simulink model "a_LS_model"  (R2023b)
settings: Solver=VariableStepAuto  StartTime=0.0  StopTime=5  RelTol=1e-3
PreLoadFcn:
  | %% Model component value calculations with holder values.
  | clear;
  | disp('PreLoaded holder values run model to apply entered T&S values ')
  | 
  | Re = [1, 1]; % The DC resistance of the Voice coil [ohm].
  | 
  | Le = [1, 1]; % The voice coil inductance [H]
  | 
  | Mms = [1, 1]; % Mass of the coil and diaphragm [Kg]
  | 
  | Sd = [1, 1] * 1e-4; % Area of diaphragm [m^2]
  | 
  | Bl = [1, 1]; % The product of magnetic flux density i.e., Force Factor
  | 
  | Vb = [1, 1];
  | 
  | fs = [1, 1];
  | 
  | Qes = [1, 1];
  | 
  | Qms = [1, 1];
  | 
  | Qts = [1, 1];
  | 
  | SweepStart_W_S = 1;
  | SweepEnd_W_S = 1;
  | SweepDuration_W_S = 1;
  | FS = 44100;
  | Qb = 0.707; % Total quality factor
  | 
  | % Constants
  | c = 340; % Speed of sound in m/s
  | rho = 1.2; % Density of air [kg/m^3]
  | r=1; % Distance for farfield calculations
  | wOffset = 0; % Driver offset for fafield calculations not used in this version
  | tOffset = 0;
  | dt=1/FS; % Time step
  | for n = 1:2
  |     alpha(n) = (Qb^2 - Qts(n)^2) / Qts(n)^2;
  |     Rms(n) = (2 * pi * fs(n) * Mms(n)) / Qms(n);
  |     Cms(n) = 1 / (4 * pi^2 * fs(n)^2 * Mms(n));
  |     Vas(n) = rho * c * Sd(n)^2 * Cms(n);
  | end
  | 
  | QB = sqrt(alpha(1) + 1) * Qts; % Electroacoustics Lecture 4 page 21
  | 
  | for n = 1:2
  |     r = 0.1;
  |     Cab(n) = Vb(n) / (rho * c^2); % Box volume acoustic compliance
  |     a(n) = sqrt(Sd(n) / pi);
  |     a(n) = 0.85;
  | 
  |     % Zc(n) = ((rho * c) / Sd(n)) * c; % from grain42n
  |     Mad(n) = (8 * rho) / (5 * (pi^2) * a(n)); % Mad (acoustic mass)
  |     Mar(n) = rho * ((a(n) * r) / Sd(n)); % from grain42n
  |     Mad(n) = Mar(n);
  | 
  |     Ras(n) = (rho * c) / (pi * (a(n)^2)); % Ras (acoustic resistance), Beranek page 820/ grain42-page 19
  |     Lem(n) = Bl(n)^2 * Cms(n); % Lem (driver's compliane in electrical domain)
  |     Rem(n) = Bl(n)^2 / Rms(n); % Rem (driver's equivalent mechanical resistance)
  |     Cem(n) = Mms(n) / (Bl(n)^2); % Cem (driver's mass in Electrical domain) from grain41en
  | 
  | 
  | 
  |     Rer(n) = (Bl(n) / Sd(n))^2 * (1 / Ras(n)); % Rea (acoustical resistance) In Electrical
  |     Leb(n) = (Bl(n) / Sd(n))^2 * Cab(n); % Lea (acoustical complance) grain42-page 19
  | 
  |     Cer(n) = (Sd(n) / Bl(n))^2 * Mar(n); % (acoustical mass) in Electrical Domain (front)
  |     Ced(n) = (Sd(n) / Bl(n))^2 * Mad(n); %(acoustical mass) in Electrical Domain (back)
  | end
  | 
  | H_prev = complex(ones(512,1));
  | H_Bt = complex(zeros(512,1));
  | tweeterHz = double(0);
  | 
  | mex mexFilter.c
  | mex mexParaFilter.c
  | mex ohmsCalc.c
InitFcn:
  | Re = [str2double(get_param('a_LS_model/T&S Values', 'W_Re')), str2double(get_param('a_LS_model/T&S Values', 'T_Re'))]; % DC resistance of the Voice coil [ohm].
  | Le = [str2double(get_param('a_LS_model/T&S Values', 'W_Le')), str2double(get_param('a_LS_model/T&S Values', 'T_Le'))] * 1e-3; % Voice coil inductance [H]
  | Mms = [str2double(get_param('a_LS_model/T&S Values', 'W_Mms')), str2double(get_param('a_LS_model/T&S Values', 'T_Mms'))] * 1e-3; % Mass of the coil and diaphragm [Kg]
  | Sd = [str2double(get_param('a_LS_model/T&S Values', 'W_Sd')), str2double(get_param('a_LS_model/T&S Values', 'T_Sd'))] * 1e-4; % Area of diaphragm [m^2]
  | Bl = [str2double(get_param('a_LS_model/T&S Values', 'W_Bl')), str2double(get_param('a_LS_model/T&S Values', 'T_Bl'))]; % Magnetic flux density product (Force Factor)
  | Vb = [str2double(get_param('a_LS_model/T&S Values', 'Vb')), str2double(get_param('a_LS_model/T&S Values', 'Vb'))];
  | fs = [str2double(get_param('a_LS_model/T&S Values', 'W_fs')), str2double(get_param('a_LS_model/T&S Values', 'T_fs'))];
  | Cms = [str2double(get_param('a_LS_model/T&S Values', 'W_Cms')), str2double(get_param('a_LS_model/T&S Values', 'W_Cms'))];
  | Qes = [str2double(get_param('a_LS_model/T&S Values', 'W_Qes')), str2double(get_param('a_LS_model/T&S Values', 'T_Qes'))];
  | Qms = [str2double(get_param('a_LS_model/T&S Values', 'W_Qms')), str2double(get_param('a_LS_model/T&S Values', 'T_Qms'))];
  | Qts = [str2double(get_param('a_LS_model/T&S Values', 'W_Qts')), str2double(get_param('a_LS_model/T&S Values', 'T_Qts'))];
  | 
  | % Load additional parameters
  | SweepStart_W_S = str2double(get_param('a_LS_model/Subsystem4', 'SweepStart'));
  | SweepEnd_W_S = str2double(get_param('a_LS_model/Subsystem4', 'SweepStop'));
  | SweepDuration_W_S = str2double(get_param('a_LS_model/Subsystem4', 'SweepTime'));
  | 
  | 
  | FS = 44100;
  | 
  | % Constants
  | c = 343; % Speed of sound in m/s
  | rho = 1.2; % Density of air [kg/m^3]
  | wOffset = str2double(get_param('a_LS_model/Subsystem1', 'distW'));
  | tOffset = str2double(get_param('a_LS_model/Subsystem1', 'distT'));
  | dt=1/FS; %time step
  | 
  | Vas(1) = rho * c * Sd(1)^2 * Cms(1);
  | 
  | for n = 1:2
  |     if n == 1
  |      fsBx = fs(1) *(Vas(1)/Vb(1)+1)^(1/2);
  |      aV = Vas(1) / Vb(1);
  |      Qb(n) = Qts(n) * sqrt(1 + aV);
  |      Rms(n) = (2 * pi * fs(n) * Mms(n)) / Qms(n);
  |      Cms(n) = 1 / ((2 * pi * fs(n))^2 * Mms(n));
  |      CmsBx = 1 / ((2 * pi * fsBx)^2 * Mms(n));
  |      QmsBx =  (2*pi*fsBx*Mms(1))/Rms(1);
  |      RmsBx = (2 * pi * fsBx * Mms(n)) / (QmsBx);
  |     elseif n == 2
  | 
  |      Cms(n) = 1 / ((2 * pi * fs(n))^2 * Mms(n));
  |      Rms(n) = (2 * pi * fs(n) * Mms(n)) / Qms(n);
  |      Vas(n) = rho * c * Sd(n)^2 * Cms(n);
  | 
  |     end
  |    alpha(n) = (Qb^2 - Qts(n)^2) / Qts(n)^2;
  | 
  | end
  | 
  | QB = sqrt(alpha(1) + 1) * Qts; % Lecture 4 page 21
  | 
  | for n = 1:2
  |     r = 0.1;
  |     Cab(n) = Vb(n) / (rho * c^2); % Box volume acoustic compliance
  |     a(n) = sqrt(Sd(n) / pi);
  |     Mad(n) = (8 * rho) / (5 * (pi^2) * a(n)); % Mad (acoustic mass)
  |     Mar(n) = rho * ((a(n) * r) / Sd(n));
  |     Ras(n) = (rho * c) / (pi * (a(n)^2)); % Ras (acoustic resistance), Beranek page 820/ grain42-page 19
  | 
  |     Lem(n) = (Bl(n)^2) * (Cms(n)); %driver compliance in electrical Domain
  |     Rem(n) = (Bl(n)^2) / Rms(n); % mechanical resistance)
  |     Cem(n) = Mms(n) / (Bl(n)^2); % mass in electical domain)
  | 
  |     Leb(n) = (Bl(n) / Sd(n))^2 * Cab(n); % Lea (acoustical compliance)
  |     Rer(n) = (Bl(n) / Sd(n))^2 * 1 / Ras(n); % Rea (acoustical resistance)
  |     Cer(n) = (Sd(n) / Bl(n))^2 * Mar(n); % Cea (acoustical mass in electrical domain Front)
  |     Ced(n) = (Sd(n) / Bl(n))^2 * Mad(n); % (acoustical mass in ED back)
  | end
  | mex mexFilter.c
  | mex mexParaFilter.c
  | mex ohmsCalc.c
StartFcn:
  | %% Model Component Value Calculations beta
  | close all;
  | 
  | disp('Thiele and Small Parameters Loaded');
  | disp('Loudspeaker Simulation Running...');
  | 
  | % Load parameters from the mask
  | Box_plot_flag = get_param('a_LS_model/T&S Values', 'Box_Plot');
  | Combo_plot_flag = get_param('a_LS_model/T&S Values', 'DSP_Plot');
  | wImpedance_plot_flag = get_param('a_LS_model/T&S Values', 'wImpedance_Plot');
  | tImpedance_plot_flag = get_param('a_LS_model/T&S Values', 'tImpedance_Plot');
  | Re = [str2double(get_param('a_LS_model/T&S Values', 'W_Re')), str2double(get_param('a_LS_model/T&S Values', 'T_Re'))]; % DC resistance of the Voice coil [ohm].
  | Le = [str2double(get_param('a_LS_model/T&S Values', 'W_Le')), str2double(get_param('a_LS_model/T&S Values', 'T_Le'))] * 1e-3; % Voice coil inductance [H]
  | Mms = [str2double(get_param('a_LS_model/T&S Values', 'W_Mms')), str2double(get_param('a_LS_model/T&S Values', 'T_Mms'))] * 1e-3; % Mass of the coil and diaphragm [Kg]
  | Sd = [str2double(get_param('a_LS_model/T&S Values', 'W_Sd')), str2double(get_param('a_LS_model/T&S Values', 'T_Sd'))] * 1e-4; % Area of diaphragm [m^2]
  | Bl = [str2double(get_param('a_LS_model/T&S Values', 'W_Bl')), str2double(get_param('a_LS_model/T&S Values', 'T_Bl'))]; % Magnetic flux density product (Force Factor)
  | Vb = [str2double(get_param('a_LS_model/T&S Values', 'Vb')), str2double(get_param('a_LS_model/T&S Values', 'Vb'))];
  | fs = [str2double(get_param('a_LS_model/T&S Values', 'W_fs')), str2double(get_param('a_LS_model/T&S Values', 'T_fs'))];
  | Cms = [str2double(get_param('a_LS_model/T&S Values', 'W_Cms')), str2double(get_param('a_LS_model/T&S Values', 'W_Cms'))];
  | Qes = [str2double(get_param('a_LS_model/T&S Values', 'W_Qes')), str2double(get_param('a_LS_model/T&S Values', 'T_Qes'))];
  | Qms = [str2double(get_param('a_LS_model/T&S Values', 'W_Qms')), str2double(get_param('a_LS_model/T&S Values', 'T_Qms'))];
  | Qts = [str2double(get_param('a_LS_model/T&S Values', 'W_Qts')), str2double(get_param('a_LS_model/T&S Values', 'T_Qts'))];
  | 
  | % Load additional parameters
  | SweepStart_W_S = str2double(get_param('a_LS_model/Subsystem4', 'SweepStart'));
  | SweepEnd_W_S = str2double(get_param('a_LS_model/Subsystem4', 'SweepStop'));
  | SweepDuration_W_S = str2double(get_param('a_LS_model/Subsystem4', 'SweepTime'));
  | 
  | figSaveFolder = get_param('a_LS_model/Teensy Script', 'figSaveFolder');
  | 
  | FS = 44100;
  | 
  | % Constants
  | c = 343; % Speed of sound in m/s
  | rho = 1.2; % Density of air [kg/m^3]
  | wOffset = str2double(get_param('a_LS_model/Subsystem1', 'distW'));
  | tOffset = str2double(get_param('a_LS_model/Subsystem1', 'distT'));
  | dt=1/FS; %time step
  | 
  | Vas(1) = rho * c * Sd(1)^2 * Cms(1);
  | 
  | for n = 1:2
  |     if n == 1
  |      fsBx = fs(1) *(Vas(1)/Vb(1)+1)^(1/2);
  |      aV = Vas(1) / Vb(1);
  |      Qb(n) = Qts(n) * sqrt(1 + aV);
  |      Rms(n) = (2 * pi * fs(n) * Mms(n)) / Qms(n);
  |      Cms(n) = 1 / ((2 * pi * fs(n))^2 * Mms(n));
  |      CmsBx = 1 / ((2 * pi * fsBx)^2 * Mms(n));
  |      QmsBx =  (2*pi*fsBx*Mms(1))/Rms(1);
  |      RmsBx = (2 * pi * fsBx * Mms(n)) / (QmsBx);
  |     elseif n == 2
  | 
  |      Cms(n) = 1 / ((2 * pi * fs(n))^2 * Mms(n));
  |      Rms(n) = (2 * pi * fs(n) * Mms(n)) / Qms(n);
  |      Vas(n) = rho * c * Sd(n)^2 * Cms(n);
  | 
  |     end
  |    alpha(n) = (Qb^2 - Qts(n)^2) / Qts(n)^2;
  | 
  | end
  | 
  | QB = sqrt(alpha(1) + 1) * Qts; % Lecture 4 page 21
  | 
  | for n = 1:2
  |     r = 0.1;
  |     Cab(n) = Vb(n) / (rho * c^2); % Box volume acoustic compliance
  |     a(n) = sqrt(Sd(n) / pi);
  |     Mad(n) = (8 * rho) / (5 * (pi^2) * a(n)); % Mad (acoustic mass)
  |     Mar(n) = rho * ((a(n) * r) / Sd(n));
  |     Ras(n) = (rho * c) / (pi * (a(n)^2)); % Ras (acoustic resistance), Beranek page 820/ grain42-page 19
  | 
  |     Lem(n) = (Bl(n)^2) * (Cms(n)); %driver compliance in electrical domain
  |     Rem(n) = (Bl(n)^2) / Rms(n); % mechanical resistance in ED
  |     Cem(n) = Mms(n) / (Bl(n)^2); %moving mass in ED
  | 
  |     Leb(n) = (Bl(n) / Sd(n))^2 * Cab(n); % Lea (acoustical compliance in ED)
  |     Rer(n) = (Bl(n) / Sd(n))^2 * 1 / Ras(n); % Rea (acoustical resistance)
  |     Cer(n) = (Sd(n) / Bl(n))^2 * Mar(n); % (acoustical mass in ED front)
  |     Ced(n) = (Sd(n) / Bl(n))^2 * Mad(n); % (acoustical mass in ED back)
  | end
  | 
  | % Low-end box response plotting
  | for n = 1:2
  |     Cas(n) = Vas(n) / (rho * c^2);
  |     W0(n) = 1 / (sqrt((Mms(n)) / Sd(n)^2 * ((Cas(n) * Cab(n)) / (Cas(n) + Cab(n)))));
  |     f = 1:512;
  |     w = 2 * pi * f;
  |     k = w / c;
  | 
  |     if strcmp(Box_plot_flag, 'on')
  |         Hb = w.^2 ./ (w.^2 - (W0(1)^2) - 1j * (W0(1) / Qb(1)) * w);
  |         figure(3);
  |         semilogx(f, 20 * log10(abs(Hb)), 'r-', 'LineWidth', 2, 'DisplayName', 'Current');
  |         hold on;
  | 
  |         legend('show', 'Location', 'southeast');
  |         grid on;
  |         hold off;
  |         ylabel('Magnitude [dB]');
  |         xlim([20 600]);
  |         ylim([-20 5]);
  |         title('Low-end box response');
  |         xticks([20 62.5 125 250 500]);
  |         xticklabels({'20', '62.5', '125', '250', '500'});
  |         xlabel('Frequency Hz');
  | 
  |         if strcmp(get_param('a_LS_model/Teensy Script', 'saveFigs'),"on")
  | 
  |           if ~exist(figSaveFolder, 'dir')
  | 
  |                mkdir(figSaveFolder);
  | 
  |           end
  |             saveas(gcf,fullfile(figSaveFolder,[figSaveFolder,'_boxResponse.png']));
  |         end
  | 
  |     end
  | end
  | 
  | % PARAMETRIC EQ
  | if strcmp(Combo_plot_flag, 'on')
  | 
  |     Hb = w.^2 ./ (w.^2 - (W0(1)^2) - 1j * (W0(1) / Qb(1)) * w);
  | 
  |     fs = 44100;
  |     Numband = 6;
  | 
  |     V0 = zeros(Numband, 1);
  |     V0_peq = zeros(Numband, 1);
  |     K = zeros(Numband, 1);
  |     fc = zeros(Numband, 1);
  |     BWp = zeros(Numband, 1);
  |     BW = zeros(Numband, 1);
  |     N = zeros(Numband, 1);
  |     w0 = zeros(Numband, 1);
  |     gain = zeros(Numband, 1);
  |     H = complex(ones(22500, 1));
  |     H_temp = complex(ones(22500, Numband));
  | 
  | % Load filter parameters
  | 
  | gain(1) = str2double(get_param('a_LS_model/Subsystem', 'GdB1'));
  | gain(2) = str2double(get_param('a_LS_model/Subsystem', 'GdB2'));
  | gain(3) = str2double(get_param('a_LS_model/Subsystem', 'GdB3'));
  | gain(4) = str2double(get_param('a_LS_model/Subsystem', 'GdB4'));
  | gain(5) = str2double(get_param('a_LS_model/Subsystem', 'GdB5'));
  | gain(6) = str2double(get_param('a_LS_model/Subsystem', 'GdB6'));
  | 
  | fc(1) = str2double(get_param('a_LS_model/Subsystem', 'FC1'));
  | fc(2) = str2double(get_param('a_LS_model/Subsystem', 'FC2'));
  | fc(3) = str2double(get_param('a_LS_model/Subsystem', 'FC3'));
  | fc(4) = str2double(get_param('a_LS_model/Subsystem', 'FC4'));
  | fc(5) = str2double(get_param('a_LS_model/Subsystem', 'FC5'));
  | fc(6) = str2double(get_param('a_LS_model/Subsystem', 'FC6'));
  | 
  | BWp(1) = str2double(get_param('a_LS_model/Subsystem', 'BW1'));
  | BWp(2) = str2double(get_param('a_LS_model/Subsystem', 'BW2'));
  | BWp(3) = str2double(get_param('a_LS_model/Subsystem', 'BW3'));
  | BWp(4) = str2double(get_param('a_LS_model/Subsystem', 'BW4'));
  | BWp(5) = str2double(get_param('a_LS_model/Subsystem', 'BW5'));
  | BWp(6) = str2double(get_param('a_LS_model/Subsystem', 'BW6'));
  | 
  | Filt=zeros(Numband,4);
  | b0=double(0);
  | b1=double(0);
  | b2=double(0);
  | a0=double(0);
  | a1=double(0);
  | a2=double(0);
  | 
  | for i=1:Numband
  | 
  | Filt(i,1)= gain(i);
  | Filt(i,2)=fc(i);
  | Filt(i,3)=BWp(i);
  | Filt(i,4)=BWp(i)*gain(i);
  | end
  | 
  | minFc=min(Filt(1:end,2));
  | maxFc=max(Filt(1:end,2));
  | 
  | 
  | for i=1:Numband
  | V0(i)= 10^(Filt(i,1)/20);%For shelving filters
  |     K(i)= tan ((pi*fc(i))/fs);
  | 
  |     V0_peq(i)=Filt(i,1);%For peaking filter
  |     w0(i) = Filt(i,2)/(fs/2);
  |     N=double(2);
  | 
  | 
  | 
  |     BW(i)=(Filt(i,2)*Filt(i,3))/100;%percentage of fc to Hz
  |     BW(i)=BW(i)/(fs/2);
  | 
  | end
  | 
  | [B,A] = designParamEQ(2,V0_peq',w0', BW','Orientation','row');
  | 
  | a0=1;
  | for i=1:Numband
  | 
  | 
  |    if Filt(i,2) ==minFc && V0(i)>0
  |       %Low Shelf Boost
  |       b0 = ((1)+(sqrt(2*V0(i))*K(i))+V0(i)*K(i)^2) / ((1)+(sqrt(2)*K(i))+K(i)^2);
  |       b1 = ((2)*(V0(i)*(K(i)^2)-1)) / ((1)+(sqrt(2)*K(i))+K(i)^2);
  |       b2 = ((1)-(sqrt(2*V0(i))*K(i))+V0(i)*K(i)^2) / ((1)+(sqrt(2)*K(i))+K(i)^2);
  |       a1 =  ((2)*((K(i)^2)-1)) / ((1)+(sqrt(2)*K(i))+K(i)^2);
  |       a2 = ((1)-sqrt(2)*K(i)+K(i)^2) / ((1)+(sqrt(2)*K(i))+K(i)^2);
  | 
  |       B(i,:)=[b0,b1,b2];
  |       A(i,:)=[a0,a1,a2];
  | 
  |    elseif Filt(i,2) == minFc && V0(i)<0
  |       %Low Shelf Cut
  | 
  |       b0=(V0(i)*(1+sqrt(2)*K(i)+K(i)^2)) / (V0(i)+sqrt(2*V0(i))*K(i)+K(i)^2);
  |       b1=(2*V0(i)*(K(i)^2-1)) / (V0(i)+sqrt(2*V0(i))*K(i)+K(i)^2);
  |       b2=(V0(i)*(1-sqrt(2)*K(i)+K(i)^2)) / (V0(i)+sqrt(2*V0(i))*K(i)+K(i)^2);
  |       a1=(2*(K(i)^2-V0(i))) / (V0(i)+sqrt(2*V0(i))*K(i)+K(i)^2);
  |       a2=(V0(i)-sqrt(2*V0(i))*K(i)+K(i)^2) / (V0(i)+sqrt(2*V0(i))*K(i)+K(i)^2);
  | 
  |       B(i,:)=[b0,b1,b2];
  |       A(i,:)=[a0,a1,a2];
  | 
  | 
  |    elseif Filt(i,2) ==maxFc && V0(i)>0
  |       % High Shelf Boost
  |       b0 = (V0(i)+sqrt(2*V0(i))*K(i)+K(i)^2) /(1+sqrt(2)*K(i)+K(i)^2);
  |       b1= (2*(K(i)^2-V0(i))) / (1+sqrt(2)*K(i)+K(i)^2);
  |       b2=  (V0(i)-sqrt(2*V0(i))*K(i)+K(i)^2) / (1+sqrt(2)*K(i)+K(i)^2);
  |       a1= (2*(K(i)^2-1)) / (1+(sqrt(2)*K(i))+K(i)^2);
  |       a2= (1-(sqrt(2)*K(i))+K(i)^2) / (1+(sqrt(2)*K(i))+K(i)^2);
  | 
  |       B(i,:)=[b0,b1,b2];
  |       A(i,:)=[a0,a1,a2];
  | 
  |     elseif Filt(i,2) == maxFc && V0(i)<0
  |        %High Shelf Cut
  | 
  |         b0=(V0(i)*(1+sqrt(2)*K(i)+K(i)^2)) / (1+sqrt(2*V0(i))*K(i)+V0(i)*K(i)^2);
  |         b1=(2*V0(i)*(K(i)^2-1)) / (1+sqrt(2*V0(i))*K(i)+V0(i)*K(i)^2);
  |         b2=(V0(i)*(1-sqrt(2)*K(i)+K(i)^2)) / (1+sqrt(2*V0(i))*K(i)+V0(i)*K(i)^2);
  |         a1=(2*(V0(i)*K(i)^2-1)) / (1+sqrt(2*V0(i))*K(i)+V0(i)*K(i)^2);
  |         a2=(1-sqrt(2*V0(i))*K(i)+V0(i)*K(i)^2) / (1+sqrt(2*V0(i))*K(i)+V0(i)*K(i)^2);
  | 
  |         B(i,:)=[b0,b1,b2];
  |         A(i,:)=[a0,a1,a2];
  | 
  |         end
  | end
  | 
  | H=complex(ones(22500));
  | for n=1:6
  | 
  | [H_temp(1:end,n),w] = freqz(B(n,1:end),A(n,1:end),22500);
  | 
  | H=H.*H_temp(1:end,n);
  | end
  | forestGreen = [34/255, 139/255, 34/255];
  | H_trunc=H(1:512);
  | H_combine=H_trunc.*Hb;
  | f=1:512;
  |         figure(4)
  |         semilogx(f, 20 * log10(abs(Hb)), 'r-', 'LineWidth', 2, 'DisplayName', 'Box');
  | 
  |         hold on
  |         semilogx(f, 20 * log10(abs(H_combine)),'Color',forestGreen,'LineStyle', '--', 'LineWidth', 2, 'DisplayName', 'Box & DSP');
  | 
  |         xlabel('Frequency (Hz)')
  |         ylabel('Magnitude (dB)')
  |         title('Magnitude Response')
  | 
  | 
  | legend('show', 'Location', 'southeast');
  | grid on
  | xlim([20 550])
  | ylim([-20 5])
  | title('Low end box and DSP combined response')
  | xticks([(20) 62.5 125 250 500 ])
  | xticklabels({'20','62.5','125','250','500'})
  | xlabel('Frequency Hz');
  | hold off
  | if strcmp(get_param('a_LS_model/Teensy Script', 'saveFigs'),"on")
  | 
  |     if ~exist(figSaveFolder, 'dir')
  | 
  |                mkdir(figSaveFolder);
  | 
  |     end
  | 
  |     saveas(gcf,fullfile(figSaveFolder,[figSaveFolder,'_boxAndDsp.png']));
  | 
  | end
  | 
  | end
  | 
  | %% IMPEDANCES
  | %Woofer
  | if strcmp(wImpedance_plot_flag, "on")
  | frq = logspace(log10(20), log10(20000), 512);
  | w = 2 * pi * frq;
  | 
  | 
  | %Empirical Le rise correction factor
  | %Various attempts for HF accuracy
  | %{
  | N=length(w);
  | ZL = 1j.*w.*Le(1);
  | 
  | D =  sum(log(w).^2) - ((1/N) * sum(log(w)))^2 + (N * (pi/2)^2);
  | a =  sum(log(abs(ZL)).*log(w)) -(1/N)*sum(log(abs(ZL))).*sum(log(w))...
  |     +(pi/2).* sum(angle(ZL));
  | n = (1/D)*a;
  | LN_K = (1/N) * (sum(log(abs(ZL))) - n *sum(log(w)));
  | K = (exp(LN_K));
  | Ls = K .* (w.^n-1) .* sin((n.*pi) / 2)*1e-3;
  | Rs = K .* (w.^n) .* cos((n.*pi) / 2);
  | %}
  | R2p = Re(1);
  | L2p = Le(1);
  | 
  | %Zemp = 1./((1./(1j .* w .* Le(1))) + (1./(R2p+(1j.*w.*L2p))));
  | %Zemp2 = (R2p.*1j.*w.*L2p)./(R2p+(1j.*w.*L2p));
  | Zemp3 = (1j * w .* Le(1)) + ((R2p*(1j*w.*L2p)) / (R2p+(1j*w.*L2p)));
  | Z_ElectricalW =  Re(1) + Zemp3;
  | 
  | %CZobel Network Impedance
  | R_ZobelW = Re(1)*1.25 ;
  | Ce_ZobelW = Le(1)/(R_ZobelW^2);
  | Z_ZobelW = R_ZobelW + (1./(1j*w*Ce_ZobelW));
  | 
  | %Mechanical Impedance
  | 
  | MmsBx = Mms(1) * ((1+ (Vas(1)/Vb(1))));
  | CemBx = MmsBx / (Bl(1)^2);
  | 
  | LemBx = (Bl(1)^2) * CmsBx;
  | ResWBx = Bl(1)^2/ RmsBx;
  | ZcWMBx = 1./(1j.*w.*CemBx);
  | ZlWMBx = 1j.*w.*LemBx;
  | 
  | 
  | ResW = Bl(1)^2/ Rms(1);
  | ZcWM = 1./(1j.*w.*Cem(1));
  | ZlWM = 1j.*w.*Lem(1);
  | 
  | Z_MechanicalW = (1./ResW) +(1./ZcWM) + (1./ZlWM);
  | 
  | Z_MechanicalWBx = (1./ResWBx) +(1./ZcWM) + (1./ZlWMBx);
  | 
  | %Total Zs
  | Z_TotalW = Z_ElectricalW + (1 ./ Z_MechanicalW);
  | 
  | Z_TotalWBx = Z_ElectricalW + (1 ./ Z_MechanicalWBx);
  | 
  | Z_TotalWZobel =  (Z_ZobelW.* Z_TotalW) ./ (Z_ZobelW + Z_TotalW);
  | 
  | 
  | %Plotting
  | figure(9)
  | subplot(2,1,1)
  | 
  | semilogx(frq, abs(Z_TotalW) , 'b', 'LineWidth', 1, 'DisplayName', 'Woofer Impedance without Zobel');
  | hold on
  | semilogx(frq, abs(Z_TotalWZobel) , 'r --', 'LineWidth', 1, 'DisplayName', 'Woofer Impedance with Zobel');
  | semilogx(frq, abs(Z_TotalWBx) , 'g --', 'LineWidth', 1, 'DisplayName', 'Woofer Impedance in box');
  | 
  | 
  | hold off
  | xlabel('Frequency (Hz)');
  | ylabel('Impedance (ohms)');
  | title(sprintf('Woofer Impedance.\n Zobel Resistor: %.2f Ohm Zobel Capacitor: %.2f μF', R_ZobelW, Ce_ZobelW*1e6));
  | 
  | legend('Location', 'Best');
  | xlim([min(frq) max(frq)])
  | xticks([20 50 100 200 500 1000 2000 5000 10000 20000]);
  | xticklabels({'20','50','100','200','500','1000','2000','5000','10000','20000'});
  | 
  | subplot(2,1,2)
  | 
  | semilogx(frq, angle(Z_TotalW)*180/pi, 'r', 'LineWidth', 1, 'DisplayName', 'Woofer Phase');
  | 
  | xlabel('Frequency (Hz)');
  | ylabel('Angle (deg)');
  | title('Woofer Phase');
  | legend('Location', 'Best');
  | xlim([min(frq) max(frq)])
  | ylim([min(angle(Z_TotalW)*180/pi) max(angle(Z_TotalW)*180/pi)])
  | xticks([20 50 100 200 500 1000 2000 5000 10000 20000]);
  | 
  | if strcmp(get_param('a_LS_model/Teensy Script', 'saveFigs'),"on")
  | 
  |     if ~exist(figSaveFolder, 'dir')
  | 
  |                mkdir(figSaveFolder);
  | 
  |     end
  | 
  |     saveas(gcf,fullfile(figSaveFolder,[figSaveFolder,'_wooferImpedance.png']));
  | 
  | end
  | 
  | end
  | 
  | % Tweeter Impedance
  | if strcmp(tImpedance_plot_flag, "on")
  | 
  | %Zobel Network Impedance
  | R_ZobelT = Re(2)*1.25 ;
  | Ce_ZobelT = Le(2)/(R_ZobelT^2);
  | 
  | Z_ZobelT = R_ZobelT + (1./(1j*w*Ce_ZobelT));
  | 
  | %Empirical Electrical Impedance
  | %{
  | ZL = 1j.*w.*Le(2);
  | D =  sum(log(w).^2) - ((1/N) * sum(log(w)))^2 + (N * (pi/2)^2);
  | a =  sum(log(abs(ZL)).*log(w)) -(1/N)*sum(log(abs(ZL))).*sum(log(w))...
  |     +(pi/2).* sum(angle(ZL));
  | n = (1/D)*a;
  | LN_K = (1/N) * (sum(log(abs(ZL))) - n *sum(log(w)));
  | K = (exp(LN_K));
  | 
  | Ls=K.*(w.^n-1).*sin((n.*pi)/2);
  | Rs=K.*(w.^n).*cos((n.*pi)/2);
  | %}
  | R2p = Re(2);
  | L2p = Le(2);
  | Zemp = 1./((1./(1j .* w .* Le(2))) + (1./(R2p+(1j.*w.*L2p))));
  | Z_ElectricalT =  Re(2) + Zemp;
  | 
  | 
  | %Mechanical Impedance
  | ResT = Bl(2)^2/ Rms(2);
  | ZcTM = 1./(1j*w*Cem(2));
  | ZlTM = 1j*w*Lem(2);
  | 
  | Z_MechanicalT = (1./ResT) +(1./ZcTM) + (1./ZlTM);
  | 
  | %Total impedance with/without Zobel network
  | 
  | Z_TotalT =  Z_ElectricalT + (1 ./ Z_MechanicalT) ;
  | Z_TotalTZobel =  (Z_ZobelT.* Z_TotalT) ./ (Z_ZobelT + Z_TotalT);
  | 
  | %Impedances for Tweeter
  | figure(10)
  | subplot(2,1,1)
  | 
  | semilogx(frq, abs(Z_TotalT) , 'b', 'LineWidth', 1, 'DisplayName', 'Tweeter Impedance');
  | hold on
  | semilogx(frq, abs(Z_TotalTZobel) , 'r--', 'LineWidth', 1, 'DisplayName', 'Tweeter Impedance with Zobel');
  | hold off
  | 
  | xlabel('Frequency (Hz)');
  | ylabel('Impedance (ohms)');
  | title(sprintf('Tweeter Impedance.\n Zobel Resistor: %.2f Ohm Zobel Capacitor: %.2f μF', R_ZobelT, Ce_ZobelT*1e6));
  | legend('Location', 'Best');
  | xlim([min(frq) max(frq)])
  | ylim([min(abs(Z_TotalTZobel)-2) max(abs(Z_TotalT)+2)])
  | 
  | 
  | xticks([20 50 100 200 500 1000 2000 5000 10000 20000]);
  | xticklabels({'20','50','100','200','500','1000','2000','5000','10000','20000'});
  | xlim([min(frq) max(frq)]);
  | subplot(2,1,2)
  | semilogx(frq, angle(Z_TotalT)*180/pi, 'r', 'LineWidth', 1, 'DisplayName', 'Tweeter Phase');
  | 
  | xlabel('Frequency (Hz)');
  | ylabel('Angle (deg)');
  | title('Tweeter Phase');
  | legend('Location', 'Best');
  | xlim([min(frq) max(frq)])
  | ylim([min(angle(Z_TotalT)*180/pi) max(angle(Z_TotalT)*180/pi)])
  | xticks([20 50 100 200 500 1000 2000 5000 10000 20000]);
  | xticklabels({'20','50','100','200','500','1000','2000','5000','10000','20000'});
  | 
  | if strcmp(get_param('a_LS_model/Teensy Script', 'saveFigs'),"on")
  | 
  |     if ~exist(figSaveFolder, 'dir')
  | 
  |                mkdir(figSaveFolder);
  | 
  |     end
  | 
  |     saveas(gcf,fullfile(figSaveFolder,[figSaveFolder,'_tweeterImpedance.png']));
  | 
  | end
  | end
StopFcn:
  | disp('Simulation Ended')
undefined symbols (not defined in the file): Ced, Cem, Cer, Leb, Lem, Rem
libraries: fl_lib x32, nesl_utility x12, dspsrcs4 x1
(part 1 of 2)
settings Model: SimulationMode=accelerator  Creator=Jamie  LastModifiedBy=jamie
settings HardwareCC: ProdBitPerLong=64  ProdHWDeviceType=Intel->x86-64 (Mac OS X)

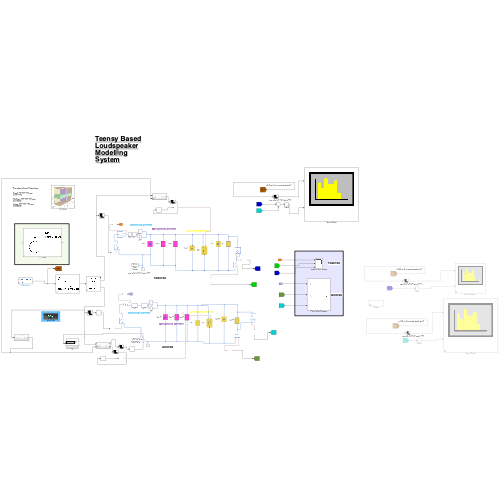
[thumbnail: Simulink's stored preview of the top-level diagram]
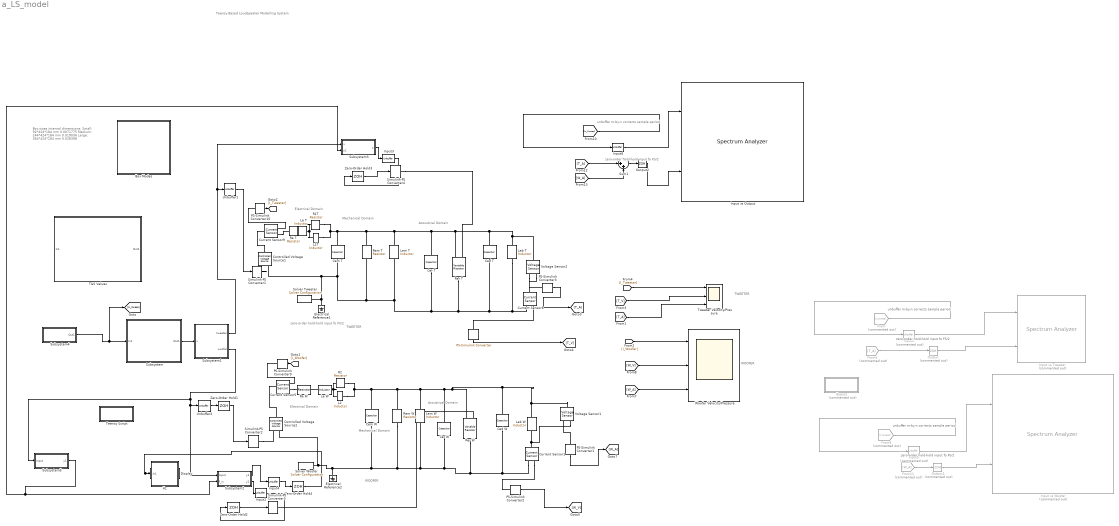
== system a_LS_model ==
  note: Teensy Based Loudspeaker Modelling System
  note: Box sizes internal dimensions:
      |
      | Small: 92*424*184 mm
      | 0.0071775
      |
      | Medium: 244*424*184 mm
      | 0.019036
      |
      | Large: 364*424*184 mm
      | 0.028398
  note: Electrical Domain
  note: Mechanical Domain
  note: Mechanical Domain
  note: WOOFER
  note: WOOFER
  note: unbuffer m-by-n corrects sample period
  note: TWEETER
  note: zero-order hold-hold input fo FS/2
  note: zero-order hold-hold input fo FS/2
  note: TWEETER
  note: Electrical Domain
  note: Acoustical Domain
  note: zero-order hold-hold input fo FS/2
  note: unbuffer m-by-n corrects sample period
  note: zero-order hold-hold input fo FS/2
  note: unbuffer m-by-n corrects sample period
  note: Acoustical Domain
  " " : nesl_utility/PS-Simulink Converter  PhysicalDomain=network_engine_domain  SubClassName=ps_output  LeftPortType=input  RightPortType=output  PseudoPeriodic=off  Frequencies=[]  VectorFormat=1-D array  Unit=1  AffineConversion=off
  Box Modes : Subsystem  mask{depth=244, height=424, width=184, vol=0.019036, boxFlag=on}
      mask prompts: depth "Depth (mm)"; height "Height (mm)"; width "Width (mm)"; vol "Volume (m^3)"; boxFlag "Calculate box modes on run (check this if using auto fig save feature)"
      mask DialogControl Control2 Prompt: Calculate volume
      mask DialogControl Control2 Callback:
      | depth= str2double(get_param('a_LS_model/Box Modes', 'depth'))*1e-3;
      | height = str2double(get_param('a_LS_model/Box Modes', 'height'))*1e-3;
      | width = str2double(get_param('a_LS_model/Box Modes', 'width'))*1e-3;
      | 
      | vol = depth*height*width;
      | 
      | set_param('a_LS_model/Box Modes','vol',num2str(vol));
      mask DialogControl Control4 Prompt: Show Box Modes
      mask DialogControl Control4 Callback:
      | depth= str2double(get_param('a_LS_model/Box Modes', 'depth'))*1e-3;
      | height = str2double(get_param('a_LS_model/Box Modes', 'height'))*1e-3;
      | width = str2double(get_param('a_LS_model/Box Modes', 'width'))*1e-3;
      | numberOfModes = 8;
      | rowNames = cell(numberOfModes,1);
      | 
      | 
      | 
      | 
      |     c = 343;
      | 
      | 
      | 
      | 
      |     depthModes = ones(numberOfModes,1);
      |     heightModes = ones(numberOfModes,1);
      |     widthModes = ones(numberOfModes,1);
      | 
      |     for i=1:numberOfModes
      | 
      |         depthModes(i)= floor((c/(2*depth))*i);
      |         heightModes(i) = floor((c/(2*height))*i);
      |         widthModes (i) = floor((c/(2*width))*i);
      | 
      |     end
      | 
      | 
      |     cNames = {'Depth'; 'Height'; 'Width'};
      | 
      | 
      |     modes = [depthModes, heightModes, widthModes];
      |     found=zeros(size(modes));
      |     toFind=double(0);
      | 
      |     %loop through matrix to find duplicates
      | 
      |     for m=1:3
      |         for j =1:numberOfModes
      |             toFind=modes(j,m);
      |             for n=1:3
      |                 for i=int8(1):numberOfModes
      |                     if modes(i, n) == toFind && (i ~= j && n ~= m)
      |                         found(i,n) = modes(i,n);
      | 
      |                     end
      |                 end
      |             end
      | 
      |         end
      | 
      |     end
      | 
      | 
      |     for i =int8(1):numberOfModes
      | 
      |         rowNames {i} = sprintf('Mode %d\n (Hz)',i);
      | 
      |     end
      | 
      | 
      | 
      | 
      |     figure(12)
      |     panel1 = uipanel('Title', 'Box Modes', 'TitlePosition','centertop','Position', [0.05, 0.05, 0.5, 0.9], 'FontSize', 18,'BackgroundColor', '#FFFDD0');
      |     panel2 = uipanel('Title', 'Duplicate Modes','TitlePosition','centertop', 'Position', [0.55, 0.05, 0.4, 0.9],'FontSize', 18, 'BackgroundColor', '#FFFDD0');
      | 
      |     uitable(panel1,"Data",modes, "ColumnName",cNames, 'RowName', rowNames,'Units', 'normalized','FontSize', 18);
      | 
      | 
      | 
      |     data = found;
      | 
      |     uitable(panel2, 'Data', data, "ColumnName",cNames,'RowName',rowNames, 'Units', 'normalized','FontSize', 18);
      | 
      |    set(gcf,'Position',[10 10 1000 400])
      mask DialogControl Control3 Prompt: To use this box volume in the model copy and paste it to the T&S Parameters block
      mask Display: image('modes.png'); % Use "Edit Image" on toolstrip to change.
  Bypass : Subsystem  Commented=on  mask{bypass=off}
      mask prompts: bypass "Bypass crossover/delay (for driver response)"
      mask DialogControl DescTextVar Prompt: This bypasses the crossover/delay/gain so the tweeter and woofer responses can be seen across full frequency band
  Ced T : fl_lib/Electrical/Electrical Elements/Capacitor  c=Ced(2) F  r=0 Ohm  g=0 1/Ohm  i_specify=off  i_priority=High  i=0 A  i_nominal_specify=off  i_nominal_unit=A  i_nominal_value=1  v_specify=off  v_priority=High  v=0 V  v_nominal_specify=off  v_nominal_unit=V  v_nominal_value=1  vc_specify=off  vc_priority=High  vc=0 V  vc_nominal_specify=off  vc_nominal_unit=V  vc_nominal_value=1
  Ced W : fl_lib/Electrical/Electrical Elements/Capacitor  c=Cer(1) F  r=0 Ohm  g=0 1/Ohm  i_specify=off  i_priority=High  i=0 A  i_nominal_specify=off  i_nominal_unit=A  i_nominal_value=1  v_specify=off  v_priority=High  v=0 V  v_nominal_specify=off  v_nominal_unit=V  v_nominal_value=1  vc_specify=off  vc_priority=High  vc=0 V  vc_nominal_specify=off  vc_nominal_unit=V  vc_nominal_value=1
  Cem T : fl_lib/Electrical/Electrical Elements/Capacitor  c=Cem(2) mF  r=0 Ohm  g=0 1/Ohm  i_specify=off  i_priority=High  i=0 A  i_nominal_specify=off  i_nominal_unit=A  i_nominal_value=1  v_specify=off  v_priority=High  v=0 V  v_nominal_specify=off  v_nominal_unit=V  v_nominal_value=1  vc_specify=off  vc_priority=High  vc=0 V  vc_nominal_specify=off  vc_nominal_unit=V  vc_nominal_value=1
  Cem W : fl_lib/Electrical/Electrical Elements/Capacitor  c=Cem(1) mF  r=0 Ohm  g=0 1/Ohm  i_specify=off  i_priority=High  i=0 A  i_nominal_specify=off  i_nominal_unit=A  i_nominal_value=1  v_specify=off  v_priority=High  v=0 V  v_nominal_specify=off  v_nominal_unit=V  v_nominal_value=1  vc_specify=off  vc_priority=High  vc=0 V  vc_nominal_specify=off  vc_nominal_unit=V  vc_nominal_value=1
  Cer T : fl_lib/Electrical/Electrical Elements/Capacitor  c=Cer(2) F  r=0 Ohm  g=0 1/Ohm  i_specify=off  i_priority=High  i=0 A  i_nominal_specify=off  i_nominal_unit=A  i_nominal_value=1  v_specify=off  v_priority=High  v=0 V  v_nominal_specify=off  v_nominal_unit=V  v_nominal_value=1  vc_specify=off  vc_priority=High  vc=0 V  vc_nominal_specify=off  vc_nominal_unit=V  vc_nominal_value=1
  Cer W : fl_lib/Electrical/Electrical Elements/Capacitor  c=Cer(1) F  r=0 Ohm  g=0 1/Ohm  i_specify=off  i_priority=High  i=0 A  i_nominal_specify=off  i_nominal_unit=A  i_nominal_value=1  v_specify=off  v_priority=High  v=0 V  v_nominal_specify=off  v_nominal_unit=V  v_nominal_value=1  vc_specify=off  vc_priority=High  vc=0 V  vc_nominal_specify=off  vc_nominal_unit=V  vc_nominal_value=1
  Controlled Voltage Source1 : fl_lib/Electrical/Electrical Sources/Controlled Voltage Source
  Controlled Voltage Source2 : fl_lib/Electrical/Electrical Sources/Controlled Voltage Source
  Current Sensor{1,5,8..9} (4 alike) : fl_lib/Electrical/Electrical Sensors/Current Sensor
  Display : Display
  Electrical Reference1 : fl_lib/Electrical/Electrical Elements/Electrical Reference
  Electrical Reference2 : fl_lib/Electrical/Electrical Elements/Electrical Reference
  From : From  Commented=on  GotoTag=In_Sweep
  From11 : From  Commented=on  GotoTag=W_A
  From5 : From  Commented=on  GotoTag=T_A
  From9 : From  Commented=on  GotoTag=In_Sweep
  Hz : Subsystem
  Input vs Output : SpectrumAnalyzer  NumInputPorts=2  WindowPosition=[1.000000,76.000000,1680.000000,922.000000,]  ScopeFrameLocation=window  Method=Welch  SampleRate=48000  PlotAsTwoSidedSpectrum=off  FrequencyScale=Log  AxesScaling=Manual  FrequencySpan=Start and stop frequencies  StartFrequency=4000  StopFrequency=20e3  AveragingMethod=Exponential  ForgettingFactor=0.4  FrequencyOffset=[500]  PlotNormalTrace=off  PlotMaxHoldTrace=on  YLimits=[-40.3301749,41.95165102]  ShowLegend=on
      settings: OpenAtSimulationStart=off
  "Input vs Tweeter  " : SpectrumAnalyzer  Commented=on  NumInputPorts=2  WindowPosition=[1.000000,76.000000,1680.000000,922.000000,]  ScopeFrameLocation=window  Method=Welch  SampleRate=48000  PlotAsTwoSidedSpectrum=off  FrequencyScale=Log  AxesScaling=Manual  FrequencySpan=Start and stop frequencies  StartFrequency=4000  StopFrequency=20e3  AveragingMethod=Exponential  ForgettingFactor=0.4  PlotNormalTrace=off  PlotMaxHoldTrace=on  YLimits=[-235.56274436,46.83172767]  ShowLegend=on
      settings: OpenAtSimulationStart=off
  Input vs Woofer : SpectrumAnalyzer  Commented=on  NumInputPorts=2  WindowPosition=[1.000000,76.000000,1680.000000,922.000000,]  ScopeFrameLocation=window  Method=Welch  SampleRate=48000  PlotAsTwoSidedSpectrum=off  FrequencyScale=Log  AxesScaling=Manual  FrequencySpan=Start and stop frequencies  StartFrequency=4000  StopFrequency=20e3  AveragingMethod=Exponential  ForgettingFactor=0.4  FrequencyOffset=[500]  PlotNormalTrace=off  PlotMaxHoldTrace=on  YLimits=[-193.2947565,31.72728743]  ShowLegend=on
      settings: OpenAtSimulationStart=off
  Input1 : Unbuffer  Commented=on
  Input{2..4,6} (4 alike) : Unbuffer
  Input5 : Unbuffer  Commented=on
  L1T : fl_lib/Electrical/Electrical Elements/Inductor  l=Le(2) H  r=0 Ohm  g=0 1/Ohm  i_specify=off  i_priority=High  i=0 A  i_nominal_specify=off  i_nominal_unit=A  i_nominal_value=1  v_specify=off  v_priority=High  v=0 V  v_nominal_specify=off  v_nominal_unit=V  v_nominal_value=1  i_L_specify=off  i_L_priority=High  i_L=0 A  i_L_nominal_specify=off  i_L_nominal_unit=A  i_L_nominal_value=1
  L2 : fl_lib/Electrical/Electrical Elements/Inductor  l=Le(1) H  r=0 Ohm  g=0 1/Ohm  i_specify=off  i_priority=High  i=0 A  i_nominal_specify=off  i_nominal_unit=A  i_nominal_value=1  v_specify=off  v_priority=High  v=0 V  v_nominal_specify=off  v_nominal_unit=V  v_nominal_value=1  i_L_specify=off  i_L_priority=High  i_L=0 A  i_L_nominal_specify=off  i_L_nominal_unit=A  i_L_nominal_value=1
  Le T : fl_lib/Electrical/Electrical Elements/Inductor  l=Le(2) H  r=0 Ohm  g=0 1/Ohm  i_specify=off  i_priority=High  i=0 A  i_nominal_specify=off  i_nominal_unit=A  i_nominal_value=1  v_specify=off  v_priority=High  v=0 V  v_nominal_specify=off  v_nominal_unit=V  v_nominal_value=1  i_L_specify=off  i_L_priority=High  i_L=0 A  i_L_nominal_specify=off  i_L_nominal_unit=A  i_L_nominal_value=1
  Le W : fl_lib/Electrical/Electrical Elements/Inductor  l=Le(1) H  r=0 Ohm  g=0 1/Ohm  i_specify=off  i_priority=High  i=0 A  i_nominal_specify=off  i_nominal_unit=A  i_nominal_value=1  v_specify=off  v_priority=High  v=0 V  v_nominal_specify=off  v_nominal_unit=V  v_nominal_value=1  i_L_specify=off  i_L_priority=High  i_L=0 A  i_L_nominal_specify=off  i_L_nominal_unit=A  i_L_nominal_value=1
  Leb T : fl_lib/Electrical/Electrical Elements/Inductor  l=Leb(2) mH  r=0 Ohm  g=0 1/Ohm  i_specify=off  i_priority=High  i=0 A  i_nominal_specify=off  i_nominal_unit=A  i_nominal_value=1  v_specify=off  v_priority=High  v=0 V  v_nominal_specify=off  v_nominal_unit=V  v_nominal_value=1  i_L_specify=off  i_L_priority=High  i_L=0 A  i_L_nominal_specify=off  i_L_nominal_unit=A  i_L_nominal_value=1
  Leb W : fl_lib/Electrical/Electrical Elements/Inductor  l=Leb(1) H  r=0 Ohm  g=0 1/Ohm  i_specify=off  i_priority=High  i=0 A  i_nominal_specify=off  i_nominal_unit=A  i_nominal_value=1  v_specify=off  v_priority=High  v=0 V  v_nominal_specify=off  v_nominal_unit=V  v_nominal_value=1  i_L_specify=off  i_L_priority=High  i_L=0 A  i_L_nominal_specify=off  i_L_nominal_unit=A  i_L_nominal_value=1
  Lem T : fl_lib/Electrical/Electrical Elements/Inductor  l=Lem(2) H  r=0 Ohm  g=0 1/Ohm  i_specify=off  i_priority=High  i=0 A  i_nominal_specify=off  i_nominal_unit=A  i_nominal_value=1  v_specify=off  v_priority=High  v=0 V  v_nominal_specify=off  v_nominal_unit=V  v_nominal_value=1  i_L_specify=off  i_L_priority=High  i_L=0 A  i_L_nominal_specify=off  i_L_nominal_unit=A  i_L_nominal_value=1
  Lem W : fl_lib/Electrical/Electrical Elements/Inductor  l=Lem(1) H  r=0 Ohm  g=0 1/Ohm  i_specify=off  i_priority=High  i=0 A  i_nominal_specify=off  i_nominal_unit=A  i_nominal_value=1  v_specify=off  v_priority=High  v=0 V  v_nominal_specify=off  v_nominal_unit=V  v_nominal_value=1  i_L_specify=off  i_L_priority=High  i_L=0 A  i_L_nominal_specify=off  i_L_nominal_unit=A  i_L_nominal_value=1
  Output : ZeroOrderHold  Commented=on  SampleTime=1/FS
  Output1 : ZeroOrderHold  Commented=on  SampleTime=1/FS
  Output2 : ZeroOrderHold  SampleTime=1/FS
  PS-Simulink Converter{1..3,9..10} (5 alike) : nesl_utility/PS-Simulink Converter  PhysicalDomain=network_engine_domain  SubClassName=ps_output  LeftPortType=input  RightPortType=output  PseudoPeriodic=off  Frequencies=[]  VectorFormat=1-D array  Unit=1  AffineConversion=off
  R1T : fl_lib/Electrical/Electrical Elements/Resistor  R=Re(2) Ohm  i_specify=off  i_priority=High  i=0 A  i_nominal_specify=off  i_nominal_unit=A  i_nominal_value=1  v_specify=off  v_priority=High  v=0 V  v_nominal_specify=off  v_nominal_unit=V  v_nominal_value=1
  R2 : fl_lib/Electrical/Electrical Elements/Resistor  R=Re(1) Ohm  i_specify=off  i_priority=High  i=0 A  i_nominal_specify=off  i_nominal_unit=A  i_nominal_value=1  v_specify=off  v_priority=High  v=0 V  v_nominal_specify=off  v_nominal_unit=V  v_nominal_value=1
  Re T : fl_lib/Electrical/Electrical Elements/Resistor  R=Re(2) Ohm  i_specify=off  i_priority=High  i=0 A  i_nominal_specify=off  i_nominal_unit=A  i_nominal_value=1  v_specify=off  v_priority=High  v=0 V  v_nominal_specify=off  v_nominal_unit=V  v_nominal_value=1
  Re W : fl_lib/Electrical/Electrical Elements/Resistor  R=Re(1) Ohm  i_specify=off  i_priority=High  i=0 A  i_nominal_specify=off  i_nominal_unit=A  i_nominal_value=1  v_specify=off  v_priority=High  v=0 V  v_nominal_specify=off  v_nominal_unit=V  v_nominal_value=1
  Rem T : fl_lib/Electrical/Electrical Elements/Resistor  R=Rem(2) Ohm  i_specify=off  i_priority=High  i=0 A  i_nominal_specify=off  i_nominal_unit=A  i_nominal_value=1  v_specify=off  v_priority=High  v=0 V  v_nominal_specify=off  v_nominal_unit=V  v_nominal_value=1
  Rem W : fl_lib/Electrical/Electrical Elements/Resistor  R=Rem(1) Ohm  i_specify=off  i_priority=High  i=0 A  i_nominal_specify=off  i_nominal_unit=A  i_nominal_value=1  v_specify=off  v_priority=High  v=0 V  v_nominal_specify=off  v_nominal_unit=V  v_nominal_value=1
  Rer T : fl_lib/Electrical/Electrical Elements/Variable Resistor  Rmin=0 Ohm  thermalEnable=false  thermal_mass=1 J/K  i_specify=off  i_priority=None  i=0 A  i_nominal_specify=off  i_nominal_unit=A  i_nominal_value=1  v_specify=off  v_priority=None  v=0 V  v_nominal_specify=off  v_nominal_unit=V  v_nominal_value=1  T_specify=off  T_priority=None  T=300 K  T_nominal_specify=off  T_nominal_unit=K  T_nominal_value=1
  Rer W : fl_lib/Electrical/Electrical Elements/Variable Resistor  Rmin=0 Ohm  thermalEnable=false  thermal_mass=1 J/K  i_specify=off  i_priority=None  i=0 A  i_nominal_specify=off  i_nominal_unit=A  i_nominal_value=1  v_specify=off  v_priority=None  v=0 V  v_nominal_specify=off  v_nominal_unit=V  v_nominal_value=1  T_specify=off  T_priority=None  T=300 K  T_nominal_specify=off  T_nominal_unit=K  T_nominal_value=1
  Simulink-PS Converter{1..4} (4 alike) : nesl_utility/Simulink-PS Converter  PhysicalDomain=network_engine_domain  SubClassName=ps_input  LeftPortType=input  RightPortType=output  PseudoPeriodic=off  Frequencies=[]  NoiseDistribution=none  NoiseParameters=[]  Unit=1  AffineConversion=off  FilteringAndDerivatives=zero  SimscapeFilterOrder=1  InputFilterTimeConstant=0.001  UdotUserProvided=1
  Solver Tweeter : nesl_utility/Solver Configuration  PhysicalDomain=network_engine_domain  SubClassName=solver  LeftPortType=input  RightPortType=generic  Tones=[]  Harmonics=[]  SimulateNoise=off  Profile=off  UseLocalSampling=off  EnableSwitchedLinearOptims=on  FrequencyDomain=off  UseCCode=off  RelTol=0.001  AbsTol=1e-06  MinStep=1e-09  ToWorkspace=off  RevertToSquareIcSolve=off  NumHomotopyIterations=100  PhasorMode=off  PhasorModeNumHarmonics=1  ConsistencySolver=NEWTON_FTOL  IndexReductionMethod=DerivativeReplacement  DoDC=off  ResidualTolerance=1e-09  ConsistencyTolSource=GLOBAL  ConsistencyAbsTol=0.001  ConsistencyRelTol=0.001  ConsistencyTolFactor=0.001  UseLocalSolver=off  LocalSolverChoice=NE_BACKWARD_EULER_ADVANCER  ResolveIndetEquations=on  FunctionEvalNumThread=1  LocalSolverSampleTime=0.001  DoFixedCost=off  MaxNonlinIter=3  MaxModeIter=2  ComputeImpulses=off  ImpulseIterations=2  LinearAlgebra=Sparse  LinearAlgebraNumThread=0  EquationFormulation=NE_TIME_EF  DelaysMemoryBudget=1024  AutomaticFiltering=on  FilteringTimeConstant=0.001  PartitionStorageMethod=AS_NEEDED  PartitionMemoryBudget=1024  PartitionMethod=FAST  MultibodyUseLocalSolver=off  MultibodyLocalSolverChoice=ODE1  MultibodyLocalSolverSampleTime=0.001
  "Solver Woofer " : nesl_utility/Solver Configuration  PhysicalDomain=network_engine_domain  SubClassName=solver  LeftPortType=input  RightPortType=generic  Tones=[]  Harmonics=[]  SimulateNoise=off  Profile=off  UseLocalSampling=off  EnableSwitchedLinearOptims=on  FrequencyDomain=off  UseCCode=off  RelTol=0.001  AbsTol=1e-06  MinStep=1e-09  ToWorkspace=off  RevertToSquareIcSolve=off  NumHomotopyIterations=100  PhasorMode=off  PhasorModeNumHarmonics=1  ConsistencySolver=NEWTON_FTOL  IndexReductionMethod=DerivativeReplacement  DoDC=off  ResidualTolerance=1e-09  ConsistencyTolSource=GLOBAL  ConsistencyAbsTol=0.001  ConsistencyRelTol=0.001  ConsistencyTolFactor=0.001  UseLocalSolver=off  LocalSolverChoice=NE_BACKWARD_EULER_ADVANCER  ResolveIndetEquations=on  FunctionEvalNumThread=1  LocalSolverSampleTime=0.001  DoFixedCost=off  MaxNonlinIter=3  MaxModeIter=2  ComputeImpulses=off  ImpulseIterations=2  LinearAlgebra=Sparse  LinearAlgebraNumThread=0  EquationFormulation=NE_TIME_EF  DelaysMemoryBudget=1024  AutomaticFiltering=on  FilteringTimeConstant=0.001  PartitionStorageMethod=AS_NEEDED  PartitionMemoryBudget=1024  PartitionMethod=FAST  MultibodyUseLocalSolver=off  MultibodyLocalSolverChoice=ODE1  MultibodyLocalSolverSampleTime=0.001
  Subsystem : Subsystem  mask{plotFlag=on, BW1=100.0, GdB1=2.9, FC1=78, BW2=78.150, GdB2=0.540, FC2=112, BW3=26.850, GdB3=0, FC3=3300, BW4=67.330, GdB4=0, FC4=2.000e+04, BW5=67.700, GdB5=0.13, FC5=180, BW6=89.550, GdB6=0.0, FC6=4000}
      mask prompts: plotFlag "Plot EQ response on run (needed for figure save function)"; BW1 "Band Width 1"; GdB1 "Gain 1"; FC1 "Center Frequency 1"; BW2 "Band Width 2"; GdB2 "Gain 2"; FC2 "Center Frequency 2"; BW3 "Band Width 3"; GdB3 "Gain 3"; FC3 "Center Frequency 3"; BW4 "Band Width 4"; GdB4 "Gain 4"; FC4 "Center Frequency 4"; BW5 "Band Width 5"; GdB5 "Gain 5"; FC5 "Center Frequency 5"; BW6 "Band Width 6"; GdB6 "Gain 6"; FC6 "Center Frequency 6"
      mask DialogControl DescTextVar Prompt: Highest and lowest fc will be shelving
      mask DialogControl Control2 Prompt: View EQ response
      mask DialogControl Control2 Callback:
      | fs =44100;
      | 
      | 
      | 
      | Numband = 6;
      | V0=zeros(Numband,1);
      | V0_peq=zeros(Numband,1);
      | K= zeros(Numband,1);
      | fc=zeros(Numband,1);
      | zeroLine=zeros(512,1);
      | BWp=zeros(Numband,1);
      | BW=zeros(Numband,1);
      | N=zeros(Numband,1);
      | w0=zeros(Numband,1);
      | H=complex(ones(512,1));
      | H_temp=complex(ones(512,Numband));
      | 
      | 
      | gain(1) = str2double(get_param('a_LS_model/Subsystem', 'GdB1'));
      | gain(2) = str2double(get_param('a_LS_model/Subsystem', 'GdB2'));
      | gain(3) = str2double(get_param('a_LS_model/Subsystem', 'GdB3'));
      | gain(4) = str2double(get_param('a_LS_model/Subsystem', 'GdB4'));
      | gain(5) = str2double(get_param('a_LS_model/Subsystem', 'GdB5'));
      | gain(6) = str2double(get_param('a_LS_model/Subsystem', 'GdB6'));
      | 
      | 
      | 
      | fc(1) = str2double(get_param('a_LS_model/Subsystem', 'FC1'));
      | fc(2) = str2double(get_param('a_LS_model/Subsystem', 'FC2'));
      | fc(3) = str2double(get_param('a_LS_model/Subsystem', 'FC3'));
      | fc(4) = str2double(get_param('a_LS_model/Subsystem', 'FC4'));
      | fc(5) = str2double(get_param('a_LS_model/Subsystem', 'FC5'));
      | fc(6) = str2double(get_param('a_LS_model/Subsystem', 'FC6'));
      | 
      | 
      | BWp(1) = str2double(get_param('a_LS_model/Subsystem', 'BW1'));
      | BWp(2) = str2double(get_param('a_LS_model/Subsystem', 'BW2'));
      | BWp(3) = str2double(get_param('a_LS_model/Subsystem', 'BW3'));
      | BWp(4) = str2double(get_param('a_LS_model/Subsystem', 'BW4'));
      | BWp(5) = str2double(get_param('a_LS_model/Subsystem', 'BW5'));
      | BWp(6) = str2double(get_param('a_LS_model/Subsystem', 'BW6'));
      | 
      | Filt=zeros(Numband,4);
      | b0=double(0);
      | b1=double(0);
      | b2=double(0);
      | a0=double(0);
      | a1=double(0);
      | a2=double(0);
      | 
      | for i=1:Numband
      | 
      | Filt(i,1)= gain(i);
      | Filt(i,2)=fc(i);
      | Filt(i,3)=BWp(i);
      | Filt(i,4)=BWp(i)*gain(i);
      | end
      | 
      | minFc=min(Filt(1:end,2));
      | maxFc=max(Filt(1:end,2));
      | 
      | 
      | 
      | for i=1:Numband
      | V0(i)= 10^(Filt(i,1)/20);%For shelving filters
      |     K(i)= tan ((pi*fc(i))/fs);
      | 
      |     V0_peq(i)=Filt(i,1);%For peaking filter
      |     w0(i) = Filt(i,2)/(fs/2);
      |     N=double(2);
      | 
      | 
      | 
      | 
      |     BW(i)=(Filt(i,2)*Filt(i,3))/100;%percentage of fc to Hz
      |     BW(i)=BW(i)/(fs/2);
      | 
      | end
      | 
      | [B,A] = designParamEQ(2,V0_peq',w0', BW','Orientation','row');
      | 
      | 
      | 
      | for i=1:Numband
      | 
      | 
      |         if Filt(i,2) ==minFc && V0(i)>0
      |             %Low Shelf Boost
      |             b0 = ((1)+(sqrt(2*V0(i))*K(i))+V0(i)*K(i)^2) / ((1)+(sqrt(2)*K(i))+K(i)^2);
      |             b1 = ((2)*(V0(i)*(K(i)^2)-1)) / ((1)+(sqrt(2)*K(i))+K(i)^2);
      |             b2 = ((1)-(sqrt(2*V0(i))*K(i))+V0(i)*K(i)^2) / ((1)+(sqrt(2)*K(i))+K(i)^2);
      |             a0 = 1;
      |             a1 =  ((2)*((K(i)^2)-1)) / ((1)+(sqrt(2)*K(i))+K(i)^2);
      |             a2 = ((1)-sqrt(2)*K(i)+K(i)^2) / ((1)+(sqrt(2)*K(i))+K(i)^2);
      | 
      |             B(i,:)=[b0,b1,b2];
      |             A(i,:)=[a0,a1,a2];
      | 
      | 
      |         elseif Filt(i,2) == minFc && V0(i)<0
      |             %Low Shelf Cut
      | 
      | 
      |             b0=(V0(i)*(1+sqrt(2)*K(i)+K(i)^2)) / (V0(i)+sqrt(2*V0(i))*K(i)+K(i)^2);
      |             b1=(2*V0(i)*(K(i)^2-1)) / (V0(i)+sqrt(2*V0(i))*K(i)+K(i)^2);
      |             b2=(V0(i)*(1-sqrt(2)*K(i)+K(i)^2)) / (V0(i)+sqrt(2*V0(i))*K(i)+K(i)^2);
      |             a0=1;
      |             a1=(2*(K(i)^2-V0(i))) / (V0(i)+sqrt(2*V0(i))*K(i)+K(i)^2);
      |             a2=(V0(i)-sqrt(2*V0(i))*K(i)+K(i)^2) / (V0(i)+sqrt(2*V0(i))*K(i)+K(i)^2);
      | 
      |             B(i,:)=[b0,b1,b2];
      |             A(i,:)=[a0,a1,a2];
      | 
      | 
      |         elseif Filt(i,2) ==maxFc && V0(i)>0
      |             % High Shelf Boost
      |             b0 = (V0(i)+sqrt(2*V0(i))*K(i)+K(i)^2) /(1+sqrt(2)*K(i)+K(i)^2);
      |             b1= (2*(K(i)^2-V0(i))) / (1+sqrt(2)*K(i)+K(i)^2);
      |             b2=  (V0(i)-sqrt(2*V0(i))*K(i)+K(i)^2) / (1+sqrt(2)*K(i)+K(i)^2);
      |             a0=1;
      |             a1= (2*(K(i)^2-1)) / (1+(sqrt(2)*K(i))+K(i)^2);
      |             a2= (1-(sqrt(2)*K(i))+K(i)^2) / (1+(sqrt(2)*K(i))+K(i)^2);
      | 
      |             B(i,:)=[b0,b1,b2];
      |             A(i,:)=[a0,a1,a2];
      | 
      | 
      | 
      |         elseif Filt(i,2) == maxFc && V0(i)<0
      |             %High Shelf Cut
      | 
      |             b0=(V0(i)*(1+sqrt(2)*K(i)+K(i)^2)) / (1+sqrt(2*V0(i))*K(i)+V0(i)*K(i)^2);
      |             b1=(2*V0(i)*(K(i)^2-1)) / (1+sqrt(2*V0(i))*K(i)+V0(i)*K(i)^2);
      |             b2=(V0(i)*(1-sqrt(2)*K(i)+K(i)^2)) / (1+sqrt(2*V0(i))*K(i)+V0(i)*K(i)^2);
      |             a0=1;
      |             a1=(2*(V0(i)*K(i)^2-1)) / (1+sqrt(2*V0(i))*K(i)+V0(i)*K(i)^2);
      |             a2=(1-sqrt(2*V0(i))*K(i)+V0(i)*K(i)^2) / (1+sqrt(2*V0(i))*K(i)+V0(i)*K(i)^2);
      | 
      | 
      | 
      |             B(i,:)=[b0,b1,b2];
      |             A(i,:)=[a0,a1,a2];
      | 
      | 
      | 
      | 
      | 
      | 
      |         end
      | 
      | end
      | 
      | 
      | 
      | 
      | 
      | %%
      | %%%%%%%%%%%%%%%%%%%%%%%%%%%%%%%%%%%%%%%%%%%%%%%%%%%%%%%%%%%%%%%%%%%%%%%%%%%%%%%%%%%%%%%%%%%%%%%%%%%%%%%%%%%%%%%%%%%%%%%%%
      | for n=1:Numband
      | 
      | [H_temp(1:512,n),w] = freqz(B(n,1:3),A(n,1:3));
      | 
      | 
      | 
      |  H=H.*H_temp(1:512,n);
      | 
      | 
      | 
      |  f=w/(2*pi)*fs;
      | 
      | 
      | 
      |         if n==Numband
      |         figure(1)
      |         subplot(2,1,1)
      |         assignin('base', 'H_Vector', mag2db(abs(H)));
      |         assignin('base', 'F_Vector', f);
      | 
      | 
      |         semilogx(f, zeroLine,'Color','#d3d3d3');
      |         hold on
      |         semilogx(f, mag2db(abs(H)));
      |         hold off
      | 
      |         xlabel('Frequency (Hz)')
      |         ylabel('Magnitude (dB)')
      |         title('Magnitude Response')
      |         ylim([-4 4])
      |         xlim([min(f) max(f)])
      | 
      |         xticks([20 50 100 200 500 1000 2000 5000 10000 20000]);
      |         xticklabels({'20','50','100','200','500','1000','2000','5000','10000','20000'});
      | 
      |         subplot(2,1,2)
      |         plot(w, angle(H));
      |         xlabel('Normalized Frequency (rad/sample)')
      |         ylabel('Phase (rad)')
      |         title('Phase Response')
      | 
      | 
      | 
      |         sgtitle('Parametric EQ');
      |         end
      | end
      mask DialogControl Control3 Prompt: View Box + DSP response
      mask DialogControl Control3 Callback:
      | Re = str2double(get_param('a_LS_model/T&S Values', 'W_Re')) ;
      | Le = str2double(get_param('a_LS_model/T&S Values', 'W_Le')) * 1e-3;
      | 
      | Mms = str2double(get_param('a_LS_model/T&S Values', 'W_Mms')) * 1e-3;
      | Sd = str2double(get_param('a_LS_model/T&S Values', 'W_Sd')) * 1e-4;
      | 
      | Vb = str2double(get_param('a_LS_model/T&S Values', 'Vb'));
      | Fs = str2double(get_param('a_LS_model/T&S Values', 'W_fs'));
      | Cms = str2double(get_param('a_LS_model/T&S Values', 'W_Cms'));
      | 
      | Qts = str2double(get_param('a_LS_model/T&S Values', 'W_Qts'));
      | 
      | 
      | 
      | % Constants
      | c = 343; % Speed of sound in m/s
      | rho = 1.2; % Density of air [kg/m^3]
      | 
      | Vas = rho * c * Sd^2 * Cms;
      | 
      | 
      | aV = Vas / Vb;
      | Qb = Qts * sqrt(1 + aV);
      | Cms = 1 / ((2 * pi * Fs)^2 * Mms);
      | 
      | Cab = Vb / (rho * c^2); % Box volume acoustic compliance
      | Cas = Vas / (rho * c^2);
      | 
      | 
      | % Low-end box response plotting
      | fs =44100;
      | 
      | 
      | 
      | Numband = 6;
      | V0=zeros(Numband,1);
      | V0_peq=zeros(Numband,1);
      | K= zeros(Numband,1);
      | fc=zeros(Numband,1);
      | zeroLine=zeros(512,1);
      | BWp=zeros(Numband,1);
      | BW=zeros(Numband,1);
      | N=zeros(Numband,1);
      | w0=zeros(Numband,1);
      | 
      | 
      | 
      | gain(1) = str2double(get_param('a_LS_model/Subsystem', 'GdB1'));
      | gain(2) = str2double(get_param('a_LS_model/Subsystem', 'GdB2'));
      | gain(3) = str2double(get_param('a_LS_model/Subsystem', 'GdB3'));
      | gain(4) = str2double(get_param('a_LS_model/Subsystem', 'GdB4'));
      | gain(5) = str2double(get_param('a_LS_model/Subsystem', 'GdB5'));
      | gain(6) = str2double(get_param('a_LS_model/Subsystem', 'GdB6'));
      | 
      | 
      | 
      | fc(1) = str2double(get_param('a_LS_model/Subsystem', 'FC1'));
      | fc(2) = str2double(get_param('a_LS_model/Subsystem', 'FC2'));
      | fc(3) = str2double(get_param('a_LS_model/Subsystem', 'FC3'));
      | fc(4) = str2double(get_param('a_LS_model/Subsystem', 'FC4'));
      | fc(5) = str2double(get_param('a_LS_model/Subsystem', 'FC5'));
      | fc(6) = str2double(get_param('a_LS_model/Subsystem', 'FC6'));
      | 
      | 
      | BWp(1) = str2double(get_param('a_LS_model/Subsystem', 'BW1'));
      | BWp(2) = str2double(get_param('a_LS_model/Subsystem', 'BW2'));
      | BWp(3) = str2double(get_param('a_LS_model/Subsystem', 'BW3'));
      | BWp(4) = str2double(get_param('a_LS_model/Subsystem', 'BW4'));
      | BWp(5) = str2double(get_param('a_LS_model/Subsystem', 'BW5'));
      | BWp(6) = str2double(get_param('a_LS_model/Subsystem', 'BW6'));
      | 
      | Filt=zeros(Numband,4);
      | b0=double(0);
      | b1=double(0);
      | b2=double(0);
      | a0=double(0);
      | a1=double(0);
      | a2=double(0);
      | 
      | for i=1:Numband
      | 
      | Filt(i,1)= gain(i);
      | Filt(i,2)=fc(i);
      | Filt(i,3)=BWp(i);
      | Filt(i,4)=BWp(i)*gain(i);
      | end
      | 
      | minFc=min(Filt(1:end,2));
      | maxFc=max(Filt(1:end,2));
      | 
      | 
      | 
      | for i=1:Numband
      | V0(i)= 10^(Filt(i,1)/20);%For shelving filters
      |     K(i)= tan ((pi*fc(i))/fs);
      | 
      |     V0_peq(i)=Filt(i,1);%For peaking filter
      |     w0(i) = Filt(i,2)/(fs/2);
      |     N=double(2);
      | 
      | 
      | 
      | 
      |     BW(i)=(Filt(i,2)*Filt(i,3))/100;%percentage of fc to Hz
      |     BW(i)=BW(i)/(fs/2);
      | 
      | end
      | 
      | [B,A] = designParamEQ(2,V0_peq',w0', BW','Orientation','row');
      | 
      | 
      | 
      | for i=1:Numband
      | 
      | 
      |         if Filt(i,2) ==minFc && V0(i)>0
      |             %Low Shelf Boost
      |             b0 = ((1)+(sqrt(2*V0(i))*K(i))+V0(i)*K(i)^2) / ((1)+(sqrt(2)*K(i))+K(i)^2);
      |             b1 = ((2)*(V0(i)*(K(i)^2)-1)) / ((1)+(sqrt(2)*K(i))+K(i)^2);
      |             b2 = ((1)-(sqrt(2*V0(i))*K(i))+V0(i)*K(i)^2) / ((1)+(sqrt(2)*K(i))+K(i)^2);
      |             a0 = 1;
      |             a1 =  ((2)*((K(i)^2)-1)) / ((1)+(sqrt(2)*K(i))+K(i)^2);
      |             a2 = ((1)-sqrt(2)*K(i)+K(i)^2) / ((1)+(sqrt(2)*K(i))+K(i)^2);
      | 
      |             B(i,:)=[b0,b1,b2];
      |             A(i,:)=[a0,a1,a2];
      | 
      | 
      |         elseif Filt(i,2) == minFc && V0(i)<0
      |             %Low Shelf Cut
      | 
      | 
      |             b0=(V0(i)*(1+sqrt(2)*K(i)+K(i)^2)) / (V0(i)+sqrt(2*V0(i))*K(i)+K(i)^2);
      |             b1=(2*V0(i)*(K(i)^2-1)) / (V0(i)+sqrt(2*V0(i))*K(i)+K(i)^2);
      |             b2=(V0(i)*(1-sqrt(2)*K(i)+K(i)^2)) / (V0(i)+sqrt(2*V0(i))*K(i)+K(i)^2);
      |             a0=1;
      |             a1=(2*(K(i)^2-V0(i))) / (V0(i)+sqrt(2*V0(i))*K(i)+K(i)^2);
      |             a2=(V0(i)-sqrt(2*V0(i))*K(i)+K(i)^2) / (V0(i)+sqrt(2*V0(i))*K(i)+K(i)^2);
      | 
      |             B(i,:)=[b0,b1,b2];
      |             A(i,:)=[a0,a1,a2];
      | 
      | 
      |         elseif Filt(i,2) ==maxFc && V0(i)>0
      |             % High Shelf Boost
      |             b0 = (V0(i)+sqrt(2*V0(i))*K(i)+K(i)^2) /(1+sqrt(2)*K(i)+K(i)^2);
      |             b1= (2*(K(i)^2-V0(i))) / (1+sqrt(2)*K(i)+K(i)^2);
      |             b2=  (V0(i)-sqrt(2*V0(i))*K(i)+K(i)^2) / (1+sqrt(2)*K(i)+K(i)^2);
      |             a0=1;
      |             a1= (2*(K(i)^2-1)) / (1+(sqrt(2)*K(i))+K(i)^2);
      |             a2= (1-(sqrt(2)*K(i))+K(i)^2) / (1+(sqrt(2)*K(i))+K(i)^2);
      | 
      |             B(i,:)=[b0,b1,b2];
      |             A(i,:)=[a0,a1,a2];
      | 
      | 
      | 
      |         elseif Filt(i,2) == maxFc && V0(i)<0
      |             %High Shelf Cut
      | 
      |             b0=(V0(i)*(1+sqrt(2)*K(i)+K(i)^2)) / (1+sqrt(2*V0(i))*K(i)+V0(i)*K(i)^2);
      |             b1=(2*V0(i)*(K(i)^2-1)) / (1+sqrt(2*V0(i))*K(i)+V0(i)*K(i)^2);
      |             b2=(V0(i)*(1-sqrt(2)*K(i)+K(i)^2)) / (1+sqrt(2*V0(i))*K(i)+V0(i)*K(i)^2);
      |             a0=1;
      |             a1=(2*(V0(i)*K(i)^2-1)) / (1+sqrt(2*V0(i))*K(i)+V0(i)*K(i)^2);
      |             a2=(1-sqrt(2*V0(i))*K(i)+V0(i)*K(i)^2) / (1+sqrt(2*V0(i))*K(i)+V0(i)*K(i)^2);
      | 
      | 
      | 
      |             B(i,:)=[b0,b1,b2];
      |             A(i,:)=[a0,a1,a2];
      | 
      | 
      | 
      | 
      | 
      | 
      |         end
      | 
      | end
      | 
      | 
      | 
      | 
      | 
      | %%
      | %%%%%%%%%%%%%%%%%%%%%%%%%%%%%%%%%%%%%%%%%%%%%%%%%%%%%%%%%%%%%%%%%%%%%%%%%%%%%%%%%%%%%%%%%%%%%%%%%%%%%%%%%%%%%%%%%%%%%%%%%
      | 
      |     W0 = 1 / (sqrt((Mms) / Sd^2 * ((Cas * Cab) / (Cas + Cab))));
      | 
      | 
      |     f = 1:512;
      |     w = 2 * pi * f;
      | 
      | 
      | 
      | 
      | Hb = w.^2 ./ (w.^2 - (W0^2) - 1j * (W0 / Qb) * w);
      | 
      | H = complex(ones(22500));
      | for n=1:6
      | 
      | [H_temp(1:22500,n),w] = freqz(B(n,1:3),A(n,1:3),22500);
      | 
      | H=H.*H_temp(1:end,n);
      | 
      | end
      | H_trunc=H(1:512);
      | H_combine=H_trunc.*Hb;
      | forestGreen = [34/255, 139/255, 34/255];
      | f=1:512;
      |         figure(4)
      |         semilogx(f, 20 * log10(abs(Hb)), 'r-', 'LineWidth', 2, 'DisplayName', 'Box');
      | 
      |         hold on
      |         semilogx(f, 20 * log10(abs(H_combine)),'Color',forestGreen, 'LineStyle', '--', 'LineWidth', 2, 'DisplayName', 'Box & DSP');
      | 
      |         xlabel('Frequency (Hz)')
      |         ylabel('Magnitude (dB)')
      |         title('Magnitude Response')
      | 
      | 
      | legend('show', 'Location', 'southeast');
      | grid on
      | xlim([20 550])
      | ylim([-20 5])
      | title('Low end box and DSP combined response')
      | xticks([(20) 62.5 125 250 500 ])
      | xticklabels({'20','62.5','125','250','500'})
      | xlabel('Frequency Hz');
      | hold off
      mask Display: image('parametric equalizer.jpg'); % Use "Edit Image" on toolstrip to change.
  Subsystem1 : Subsystem  mask{response=on, filter_order=4th, fc=1.474e+03, G_W=-3, G_T=0.0, distW=0.0, distT=0.500, delay=on}
      mask prompts: response "Plot frequency response on run. Needed for auto plot save function."; filter_order "2nd, 4th, or 8th Order Linkwitz Riley"; fc "Center frequency (Hz)"; G_W "Post Filter Wooofer Gain (dB)"; G_T "Post Filter Tweeter Gain (dB)"; distW "Woofer Offset (m)"; distT "Tweeter Offset (m)"; delay "Delay Plot"
      mask TypeOptions filter_order: 2nd | 4th | 8th
      mask DialogControl Control2 Prompt: View frequency response
      mask DialogControl Control2 Callback:
      | filterOrder = get_param('a_LS_model/Subsystem1', 'filter_order');
      | fc = str2double(get_param('a_LS_model/Subsystem1', 'fc'));
      | fs =44100;
      | H=zeros(512,1);
      | w=double(0);
      | 
      | w =fc/(fs/2);
      | 
      | if strcmp(filterOrder,'8th')
      | 
      |     butterOrder=4;
      | 
      | elseif strcmp(filterOrder,'4th')
      | 
      |     butterOrder=2;
      | 
      | else
      | 
      |    butterOrder=1;
      | end
      | 
      | 
      | [B_low, A_low]= butter(butterOrder, w, "low");
      | 
      | [B_high, A_high]= butter(butterOrder, w, "high");
      | 
      | 
      | 
      | 
      | 
      | 
      | 
      | 
      |         figure(2)
      |         set(gcf, 'Position', [100, 100, 800, 600]);
      | 
      |         [H_high, ~]=freqz(B_high,A_high);
      |         [H_low, w]=freqz(B_low,A_low);
      | 
      | 
      |         f=w/(2*pi)*fs;
      | 
      |         H_high_2=H_high.*H_high;
      | 
      |         H_low_2=H_low.*H_low;
      | 
      | 
      | 
      |         subplot(3,1,1)
      |         semilogx(f, mag2db(abs(H_high_2)),'b-','DisplayName', 'Second Cascade');
      |         hold on
      |         semilogx(f, mag2db(abs(H_high)),'g-', 'DisplayName', 'First Cascade');
      |         hold off
      |         xlabel('Frequency (Hz)')
      |         ylabel('Magnitude (dB)')
      |         title('Magnitude Response High Pass')
      |         ylim([-14 14])
      |         xlim([min(f) max(f)])
      | 
      |         xticks([20 50 100 200 500 1000 2000 5000 10000 20000]);
      |         xticklabels({'20','50','100','200','500','1000','2000','5000','10000','20000'});
      |         legend('show', 'Location', 'best');
      |         subplot(3,1,2)
      |         semilogx(f, mag2db(abs(H_low_2)),'b-','DisplayName', 'Second Cascade');
      |         hold on
      |         semilogx(f, mag2db(abs(H_low)),'g-','DisplayName', 'First Cascade');
      |         hold off
      |         xlabel('Frequency (Hz)')
      |         ylabel('Magnitude (dB)')
      |         title('Magnitude Response Low pass')
      |         ylim([-14 14])
      |         xlim([min(f) max(f)])
      | 
      |         xticks([20 50 100 200 500 1000 2000 5000 10000 20000]);
      |         xticklabels({'20','50','100','200','500','1000','2000','5000','10000','20000'});
      |         legend('show', 'Location', 'best');
      |         subplot(3,1,3)
      |         semilogx(f, mag2db(abs(H_low_2)),'r--','DisplayName', 'Low Pass');
      |          hold on
      |         semilogx(f, mag2db(abs(H_high_2)),'r-','DisplayName', 'High Pass');
      |         legend('show', 'Location', 'best');
      |         if double(length(B_low))==2
      | 
      |             H_low_2_inverted=H_low_2.*-1;
      |             semilogx(f, mag2db(abs(H_high_2+H_low_2_inverted)),'b-','DisplayName', 'Combined Response');
      | 
      | 
      |             hold off
      |             xlabel('Frequency (Hz)')
      |             ylabel('Magnitude (dB)')
      |             title('Magnitude Response Linkwitz-Riley 2nd Order')
      | 
      |         elseif double(length(B_low))==3
      | 
      |             semilogx(f, mag2db(abs(H_high_2+H_low_2)),'b-','DisplayName', 'Combined Response');
      | 
      | 
      |             hold off
      |             xlabel('Frequency (Hz)')
      |             ylabel('Magnitude (dB)')
      |             title('Magnitude Response Linkwitz-Riley 4th Order')
      | 
      | 
      |         else
      | 
      |             semilogx(f, mag2db(abs(H_high_2+H_low_2)),'b-','DisplayName', 'Combined Response');
      | 
      | 
      |             hold off
      |             xlabel('Frequency (Hz)')
      |             ylabel('Magnitude (dB)')
      |             title('Magnitude Response Linkwitz-Riley 8th Order')
      | 
      |         end
      | 
      |         ylim([-14 14])
      |         xlim([min(f) max(f)])
      | 
      |         xticks([20 50 100 200 500 1000 2000 5000 10000 20000]);
      |         xticklabels({'20','50','100','200','500','1000','2000','5000','10000','20000'});
      | 
      |         if strcmp(filterOrder,'4th')
      | 
      |             sgtitle('Linkwitz-Riley 4th Order Crossover');
      | 
      |         elseif strcmp(filterOrder,'8th')
      | 
      |             sgtitle('Linkwitz-Riley 8th Order Crossover');
      | 
      |         else
      | 
      |             sgtitle('Linkwitz-Riley 2nd Order Crossover');
      | 
      |         end
      mask DialogControl DescTextVar Prompt: Offset is (backwards) on the Z axis.
      mask Display: image('crossover.jpg'); % Use "Edit Image" on toolstrip to change.
  Subsystem2 : Subsystem
  Subsystem3 : Subsystem
  Subsystem4 : Subsystem  mask{SweepStart=1000, SweepStop=12000, SweepTime=5.0}
      mask prompts: SweepStart "Sweep start frequency"; SweepStop "Sweep end frequency"; SweepTime "Sweep time in seconds"
      mask Display: image('sine sweep input.jpg'); % Use "Edit Image" on toolstrip to change.
  Subsystem5 : Subsystem
  Sum1 : Sum  Inputs=|++
  T&S Values : Subsystem  mask{Vb=0.1, W_Re=3.2, T_Re=3.2, W_Le=0.97, T_Le=0.04, W_fs=53.8, T_fs=750, W_Qms=3.14, T_Qms=3.0, W_Qes=0.4, T_Qes=1.78, W_Qts=0.35, T_Qts=1.12, W_Mms=9.9, T_Mms=0.3, W_Sd=50.3, T_Sd=6.2, W_Bl=5.2, T_Bl=1.6, W_Cms=0.88, Box_Plot=on, DSP_Plot=on, wImpedance_Plot=on, tImpedance_Plot=on}
      mask prompts: Vb "Box Volume (m^3)"; W_Re "Woofer Re (Ω)"; T_Re "Tweeter Re (Ω)"; W_Le "Woofer Le (mH)"; T_Le "Tweeter Le (mH)"; W_fs "Woofer fs (Hz)"; T_fs "Tweeter fs (Hz)"; W_Qms "Woofer Qms"; T_Qms "Tweeter Qms"; W_Qes "Woofer Qes"; T_Qes "Tweeter Qes"; W_Qts "Woofer Qts"; T_Qts "Tweeter Qts"; W_Mms "Woofer Mms (g)"; T_Mms "Tweeter Mms (g)"; W_Sd "Woofer Sd (cm^3)"; T_Sd "Tweeter Sd (cm^3)"; W_Bl "Woofer Bl (Tm)"; T_Bl "Tweeter Bl (Tm)"; W_Cms "Woofer Cms (mm/N)"; Box_Plot "Low Frquency Box Plot"; DSP_Plot "Low Frequency Box Plot + DSP"; wImpedance_Plot "Woofer Impedance Plot"; tImpedance_Plot "Tweeter Impedance Plot"
      mask DialogControl Control16 Prompt: Thiele and Small Parameters
      mask DialogControl load1 Prompt: Load Woofer
      mask DialogControl save1 Prompt: Save Woofer
      mask DialogControl load2 Prompt: Load Tweeter
      mask DialogControl save2 Prompt: Save Tweeter
      mask DialogControl Control13 Prompt: Preloaded Drivers
      mask DialogControl Sig120 Prompt: Load Sig120
      mask DialogControl Sig180 Prompt: Load Sig180
      mask DialogControl Tcp4 Prompt: Load TCP 115-4
      mask DialogControl Tcp8 Prompt: Load TCP 115-8
      mask DialogControl Control13_copy Prompt: Show Plots
      mask DialogControl boxPlot Prompt: Show Box Plot
      mask DialogControl wooferZ Prompt: Show Woofer Impedance
      mask DialogControl tweeterZ Prompt: Show Tweeter Impedance
      mask DialogControl Control15 Prompt: Calculate on run. Check if using auto fig save function
      mask Display: image('$imagefile'); % Use "Edit Image" on toolstrip to change.
  Teensy Script : Subsystem  mask{savename=APresA.txt, saveFigs=on, figSaveFolder=APresA}
      mask prompts: savename "Script.txt save name"; saveFigs "Save Figures. Figures will be overwritten, folder will be created in root dir"; figSaveFolder "Figure Save Folder Name"
      mask Display: image('teensy_pic_for_mask.jpg'); % Use "Edit Image" on toolstrip to change.
  Tweeter Velocity/Pressure : Scope  NumInputPorts=3
  Unbuffer1 : Unbuffer
  Unbuffer2 : Unbuffer
  Voltage Sensor1 : fl_lib/Electrical/Electrical Sensors/Voltage Sensor
  Voltage Sensor2 : fl_lib/Electrical/Electrical Sensors/Voltage Sensor
  Woofer Velocity/Pressure : Scope  NumInputPorts=3
  Zero-Order Hold{1..4} (4 alike) : ZeroOrderHold  SampleTime=1/FS
  wires:
  Zero-Order Hold3/1 -> Simulink-PS Converter4/1
  Subsystem2/2(y2) -> Input2/1
  Zero-Order Hold1/1 -> Simulink-PS Converter2/1
  [I_Tweeter] -> Tweeter Velocity/Pressure/1
  PS-Simulink Converter9/1 -> [I_Woofer]
  Subsystem3/1(y) -> Input3/1
  Input2/1 -> Zero-Order Hold2/1
  Unbuffer2/1 -> Zero-Order Hold1/1
  Zero-Order Hold2/1 -> Simulink-PS Converter3/1
  Input3/1 -> Zero-Order Hold3/1
  [I_Woofer] -> Woofer Velocity/Pressure/1
  [W_V] -> Woofer Velocity/Pressure/2
  [T_A] -> Tweeter Velocity/Pressure/3
  PS-Simulink Converter10/1 -> [I_Tweeter]
  [T_V] -> Tweeter Velocity/Pressure/2
  [W_A] -> Woofer Velocity/Pressure/3
  From5/1 -> Output/1
  Unbuffer1/1 -> Simulink-PS Converter1/1
  Subsystem/1(Out1) -> Subsystem1/1(x)
  Subsystem2/1(y1) -> Input4/1
  Input4/1 -> Zero-Order Hold4/1
  Zero-Order Hold4/1 -> Hz/1(In1), Display/1
  Input1/1 -> "Input vs Tweeter  "/1
  From/1 -> Input1/1
  Output/1 -> "Input vs Tweeter  "/2
  " "/1 -> [T_V]
  PS-Simulink Converter3/1 -> [T_A]
  Subsystem1/1(tweeter) -> Subsystem3/1(x), Unbuffer1/1
  PS-Simulink Converter2/1 -> [W_V]
  From11/1 -> Output1/1
  Output1/1 -> Input vs Woofer/2
  From9/1 -> Input5/1
  Input5/1 -> Input vs Woofer/1
  Sum1/1 -> Output2/1
  Output2/1 -> Input vs Output/2
  Input6/1 -> Input vs Output/1
  [In_Sweep] -> Input6/1
  [T_A] -> Sum1/1
  [W_A] -> Sum1/2
  Subsystem1/2(woofer) -> Subsystem5/1(Input), Subsystem2/1(Input), Unbuffer2/1
  Subsystem5/1(y1) -> Subsystem2/2(f_in), Subsystem3/2(y1)
  PS-Simulink Converter1/1 -> [W_A]
  Subsystem4/1(Out1) -> [In_Sweep], Subsystem/1(In1)
  connections:
  PS-Simulink Converter1/LConn1 -- Voltage Sensor1/RConn1
  Simulink-PS Converter1/RConn1 -- Controlled Voltage Source1/RConn1
  Simulink-PS Converter4/RConn1 -- Rer T/LConn1
  PS-Simulink Converter10/LConn1 -- Current Sensor9/RConn1
  Simulink-PS Converter2/RConn1 -- Controlled Voltage Source2/RConn1
  Le T/LConn1 -- Re T/RConn1
  PS-Simulink Converter9/LConn1 -- Current Sensor5/RConn1
  Voltage Sensor2/RConn1 -- PS-Simulink Converter3/LConn1
  Current Sensor9/RConn2 -- Re T/LConn1
  Current Sensor9/LConn1 -- Controlled Voltage Source1/LConn1
  Controlled Voltage Source2/LConn1 -- Current Sensor5/LConn1
  Current Sensor5/RConn2 -- Re W/LConn1
  Rer W/LConn1 -- Simulink-PS Converter3/RConn1
  R1T/RConn1 -- L1T/RConn1 -- Cem T/LConn1 -- Rem T/LConn1 -- Lem T/LConn1 -- Voltage Sensor2/LConn1 -- Leb T/LConn1 -- Ced T/LConn1 -- Rer T/LConn2 -- Cer T/LConn1
  Ced T/RConn1 -- Current Sensor8/RConn2 -- Leb T/RConn1 -- Rer T/RConn1 -- Cer T/RConn1 -- Lem T/RConn1 -- Rem T/RConn1 -- Solver Tweeter/RConn1 -- Electrical Reference1/LConn1 -- Controlled Voltage Source1/RConn2 -- Cem T/RConn1
  " "/LConn1 -- Current Sensor8/RConn1
  Ced W/RConn1 -- Current Sensor1/RConn2 -- Rer W/RConn1 -- "Solver Woofer "/RConn1 -- Controlled Voltage Source2/RConn2 -- Electrical Reference2/LConn1 -- Cem W/RConn1 -- Rem W/RConn1 -- Lem W/RConn1 -- Cer W/RConn1
  L2/RConn1 -- R2/RConn1 -- Cem W/LConn1 -- Rem W/LConn1 -- Cer W/LConn1 -- Rer W/LConn2 -- Ced W/LConn1 -- Voltage Sensor1/LConn1 -- Leb W/LConn1 -- Lem W/LConn1
  Current Sensor1/RConn1 -- PS-Simulink Converter2/LConn1
  Le W/LConn1 -- Re W/RConn1
  Voltage Sensor1/RConn2 -- Current Sensor1/LConn1 -- Leb W/RConn1
  Voltage Sensor2/RConn2 -- Current Sensor8/LConn1
  Le W/RConn1 -- L2/LConn1 -- R2/LConn1
  R1T/LConn1 -- L1T/LConn1 -- Le T/RConn1
